simulink model "Controlador"  (Simulink 7.9)
settings: Solver=ode5  StartTime=0.0  StopTime=inf  RelTol=1e-3
values from neighbouring files (symbols this model uses):
  adis = [0.914511514614  0.00121885851927  2.32580878052e-05; -18.4413378208  -0.92636613517  0.000893012709119; -708.069777061  -89.1232937476  -0.938877243225]    [workspace.mat]
  bdis = [0.0778470295061 0.60373728431 237.584820105]    [workspace.mat]
  cdis = [1 0 0]    [workspace.mat]
  hdis = [-3.66524411789 2900.58437447 278392.237488]    [workspace.mat]
  kidis = -0.214176857697    [workspace.mat]
  kpdis = [2.2447842013 0.000170881301687 2.70063447362e-05]    [workspace.mat]
  tm = 0.01    [workspace.mat]
undefined symbols (not defined in the file or in its folder): National_Instruments, PCI
libraries: rtwinlib x2, simulink x1
settings Model: Creator=oscar_mau.fernandez  LastModifiedBy=automatica  SimulationMode=external
settings HardwareCC: ProdIntDivRoundTo=Zero  ProdEndianess=LittleEndian  ProdHWDeviceType=Generic->32-bit x86 compatible
settings RTWCC: SystemTargetFile=rtwin.tlc  TemplateMakefile=rtwin.tmf  Description=Real-Time Windows Target  RetainRTWFile=on  ProcessScript=rtwin_make_rtw_hook  RTWCompilerOptimization=On
settings CodeAppCC: MaxIdLength=95
settings RTWinTargetCC: TargetLibSuffix=_rtwin.lib  TargetPreCompLibLocation=C:\Archivos de programa\MATLAB\R2012a\toolbox\rtw\targets\rtwin\lib\win32  CodeReplacementLibrary=ANSI_C  CodeExecutionProfiling=off  PortableWordSizes=off  RTWinDir=C:/ARCHIV~1/MATLAB/R2012a/toolbox/rtw/targets/rtwin  TargetArch=win32  RebuildAll=on

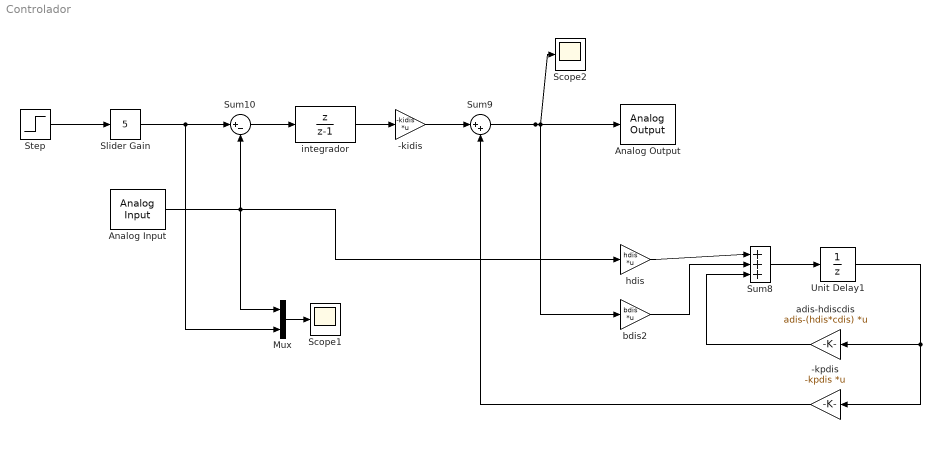
== system Controlador ==
  -kidis : Gain  Gain=-kidis  Multiplication=Matrix(K*u) (u vector)  SampleTime=tm
  -kpdis : Gain  Gain=-kpdis  Multiplication=Matrix(K*u) (u vector)  SampleTime=tm
  Analog Input : rtwinlib/Analog Input  SampleTime=tm  MaxMissedTicks=10  ShowMissedTicks=off  YieldWhenWaiting=off  DrvName=National_Instruments/PCI-6221  DrvAddress=4294967295  DrvOptions=[1 0 0 0 0]  Channels=1  RangeMode=1  VoltRange=2  DataType=1
      settings: AttributesFormatString=National Instruments\nPCI-6221 [auto]
  Analog Output : rtwinlib/Analog Output  SampleTime=tm  MaxMissedTicks=10  ShowMissedTicks=off  YieldWhenWaiting=off  DrvName=National_Instruments/PCI-6221  DrvAddress=4294967295  DrvOptions=[1 0 0 0 0]  Channels=1  RangeMode=1  VoltRange=1  InitialValue=0  FinalValue=5
      settings: AttributesFormatString=National Instruments\nPCI-6221 [auto]
  Mux : Mux  Inputs=2
  Scope1 : Scope
      settings: TimeRange=100  YMin=4.85  YMax=5.02
  Scope2 : Scope
      settings: TimeRange=100  YMin=4.85  YMax=5.02
  Slider Gain : simulink/Math Operations/Slider Gain  low=0  gain=5  high=5
  Step : Step  Time=0  SampleTime=tm
  Sum10 : Sum  Inputs=|+-  SampleTime=tm
  Sum8 : Sum  Inputs=|+++  SampleTime=tm
  Sum9 : Sum  Inputs=|++  SampleTime=tm
  Unit Delay1 : UnitDelay  SampleTime=tm
  adis-hdiscdis : Gain  Gain=adis-(hdis*cdis)  Multiplication=Matrix(K*u) (u vector)  SampleTime=tm
  bdis2 : Gain  Gain=bdis  Multiplication=Matrix(K*u) (u vector)  SampleTime=tm
  hdis : Gain  Gain=hdis  Multiplication=Matrix(K*u) (u vector)  SampleTime=tm
  integrador : DiscreteTransferFcn  Numerator=[1 0]  Denominator=[1 -1]  SampleTime=tm
  wires:
  hdis/1 -> Sum8/1
  bdis2/1 -> Sum8/2
  Sum8/1 -> Unit Delay1/1
  Unit Delay1/1 -> -kpdis/1, adis-hdiscdis/1
  adis-hdiscdis/1 -> Sum8/3
  Sum9/1 -> Analog Output/1, bdis2/1, Scope2/1
  -kidis/1 -> Sum9/1
  integrador/1 -> -kidis/1
  Sum10/1 -> integrador/1
  -kpdis/1 -> Sum9/2
  Analog Input/1 -> Sum10/2, hdis/1, Mux/1
  Step/1 -> Slider Gain/1
  Mux/1 -> Scope1/1
  Slider Gain/1 -> Sum10/1, Mux/2
